simulink model "PotholeAlertModel"  (R2025b)
settings: Solver=FixedStepAuto  StartTime=0.0  StopTime=10.0  RelTol=1e-3
libraries: simulink x2
settings Model: Creator=NSA7HC  LastModifiedBy=NSA7HC
settings OptimizationCC: DefaultParameterBehavior=Inlined  EnhancedBackFolding=on  PassReuseOutputArgsAs=Individual arguments  ZeroExternalMemoryAtStartup=off  ZeroInternalMemoryAtStartup=off  MaxStackSize=200000  OptimizeBlockOrder=speed  DifferentSizesBufferReuse=on  OptimizationCustomize=off  EfficientTunableParamExpr=on
settings DebuggingCC: ParameterTunabilityLossMsg=error
settings HardwareCC: ProdBitPerLong=64.0  ProdLargestAtomicInteger=LongLong  ProdLargestAtomicFloat=Double  ProdLongLongMode=on  ProdHWDeviceType=ARM Compatible->ARM Cortex-A (64-bit)  UseEmbeddedCoderFeatures=off
settings SFSimCC: SimCustomHeaderCode="#include \"da_connector.h\""  SimUserSources=da_connector.c  SimUserIncludeDirs=C:\Users\nsa7hc\Desktop\sdv-blueprints-fork\matlab-connector\dreamkit\c_caller  MATLABDynamicMemAlloc=off
settings RTWCC: SystemTargetFile=ert.tlc  HardwareBoard=NVIDIA Jetson  TLCOptions="-aInlineSetEventsForThisBaseRateFcn=TLC_FALSE -aSuppressMultiTaskScheduler=TLC_FALSE  -aRateBasedStepFcn=0"  TemplateMakefile=ert_default_tmf  CustomHeaderCode="#include \"da_connector.h\""  CustomInclude=C:\Users\nsa7hc\Desktop\sdv-blueprints-fork\matlab-connector\dreamkit\c_caller  CustomSource=da_connector.c  Description=Embedded Coder
settings CodeAppCC: ForceParamTrailComments=on  IgnoreCustomStorageClasses=off  OperatorAnnotations=on  SimulinkDataObjDesc=on  SFDataObjDesc=on  InsertBlockDesc=on
settings ERTTargetCC: ExtModeTransport=2.0  ExtModeStaticAlloc=on  ExtModeMexFile=ext_xcp  ExtModeIntrfLevel=Level2 - Open  SupportNonInlinedSFcns=on

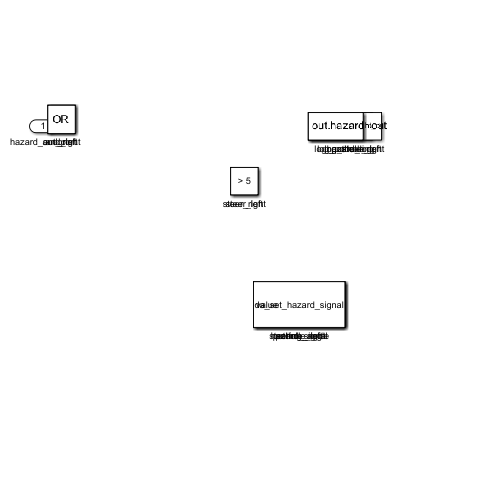
[thumbnail: Simulink's stored preview of the top-level diagram]
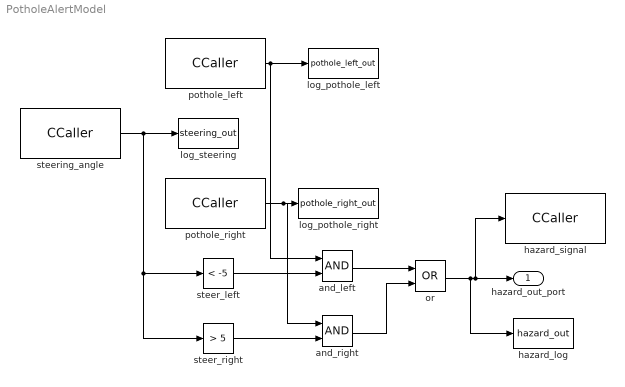
== system PotholeAlertModel ==
  and_left : Logic  AllPortsSameDT=off  OutDataTypeStr=boolean
  and_right : Logic  AllPortsSameDT=off  OutDataTypeStr=boolean
  hazard_log : ToWorkspace  VariableName=hazard_out  SaveFormat=Timeseries  SampleTime=-1
  hazard_signal : CCaller  FunctionName=da_set_hazard_signal  PortSpecificationStruct="%)30     .    * (   8    (     @         %    \"     $    !     0         %  0 \"0    $    _    07)G3F%M90  4&]R=$YA;64 4V-O<&4     26YD97@     5'EP90      4VEZ90      27-';&]B86P   X    X    !@    @    $          4    (     0    4    !         !     %    =F%L=64    .    .     8    (    !          %    \"     $    %     0         0    !0   '9A;'5E    #@   #@    &    \"     0         !0    @    !    !0    $         $     4   !);G!U=     X    X    !@    @    &          4    (     0    $    !          D    (               .    .     8    (    !          %    \"     $    '     0         0    !P   &)O;VQE86X #@   #     &    \"     0         !0    @    !     0    $         $  ! #$    .    ,     8    (    \"0(        %    \"     $    !     0         \"  $"  SampleTime=0.01
  log_pothole_left : ToWorkspace  VariableName=pothole_left_out  SaveFormat=Timeseries  SampleTime=-1
  log_pothole_right : ToWorkspace  VariableName=pothole_right_out  SaveFormat=Timeseries  SampleTime=-1
  log_steering : ToWorkspace  VariableName=steering_out  SaveFormat=Timeseries  SampleTime=-1
  or : Logic  Operator=OR  AllPortsSameDT=off  OutDataTypeStr=boolean
  pothole_left : CCaller  FunctionName=da_get_pothole_left  PortSpecificationStruct="%)30     .    & (   8    (     @         %    \"     $    !     0         %  0 \"0    $    _    07)G3F%M90  4&]R=$YA;64 4V-O<&4     26YD97@     5'EP90      4VEZ90      27-';&]B86P   X    P    !@    @    $          4    (     0    ,    !         !   P!O=70 #@   #     &    \"     0         !0    @    !     P    $         $  # &]U=  .    .     8    (    !          %    \"     $    &     0         0    !@   $]U='!U=   #@   #@    &    \"     8         !0    @    !     0    $         \"0    @               X    X    !@    @    $          4    (     0    8    !         !     &    9&]U8FQE   .    ,     8    (    !          %    \"     $    !     0         0  $ ,0    X    P    !@    @    ) @        4    (     0    $    !          (  0"  SampleTime=0.01
  pothole_right : CCaller  FunctionName=da_get_pothole_right  PortSpecificationStruct="%)30     .    & (   8    (     @         %    \"     $    !     0         %  0 \"0    $    _    07)G3F%M90  4&]R=$YA;64 4V-O<&4     26YD97@     5'EP90      4VEZ90      27-';&]B86P   X    P    !@    @    $          4    (     0    ,    !         !   P!O=70 #@   #     &    \"     0         !0    @    !     P    $         $  # &]U=  .    .     8    (    !          %    \"     $    &     0         0    !@   $]U='!U=   #@   #@    &    \"     8         !0    @    !     0    $         \"0    @               X    X    !@    @    $          4    (     0    8    !         !     &    9&]U8FQE   .    ,     8    (    !          %    \"     $    !     0         0  $ ,0    X    P    !@    @    ) @        4    (     0    $    !          (  0"  SampleTime=0.01
  steer_left : simulink/Logic and Bit Operations/Compare To Constant  relop=<  const=-5  OutDataTypeStr=boolean
  steer_right : simulink/Logic and Bit Operations/Compare To Constant  relop=>  const=5  OutDataTypeStr=boolean
  steering_angle : CCaller  FunctionName=da_get_steering_angle  PortSpecificationStruct="%)30     .    & (   8    (     @         %    \"     $    !     0         %  0 \"0    $    _    07)G3F%M90  4&]R=$YA;64 4V-O<&4     26YD97@     5'EP90      4VEZ90      27-';&]B86P   X    P    !@    @    $          4    (     0    ,    !         !   P!O=70 #@   #     &    \"     0         !0    @    !     P    $         $  # &]U=  .    .     8    (    !          %    \"     $    &     0         0    !@   $]U='!U=   #@   #@    &    \"     8         !0    @    !     0    $         \"0    @               X    X    !@    @    $          4    (     0    8    !         !     &    9&]U8FQE   .    ,     8    (    !          %    \"     $    !     0         0  $ ,0    X    P    !@    @    ) @        4    (     0    $    !          (  0"  SampleTime=0.01
  hazard_out_port : Outport
  wires:
  steer_left/1 -> and_left/2
  pothole_left/1 -> and_left/1, log_pothole_left/1
  steering_angle/1 -> steer_left/1, steer_right/1, log_steering/1
  or/1 -> hazard_signal/1, hazard_out_port/1, hazard_log/1
  pothole_right/1 -> and_right/1, log_pothole_right/1
  steer_right/1 -> and_right/2
  and_right/1 -> or/2
  and_left/1 -> or/1
